simulink model "SVPWM1"  (Simulink 9.3)
settings: Solver=ode45  StartTime=0.0  StopTime=0.2  RelTol=1e-3
libraries: powerlib x12, simulink x1
settings Model: Creator=LENOVO  LastModifiedBy=LENOVO
settings DataIOCC: SaveFormat=Dataset  SignalLoggingSaveFormat=Dataset  ReturnWorkspaceOutputs=on
settings DebuggingCC: UnderspecifiedInitializationDetection=Simplified  MergeDetectMultiDrivingBlocksExec=error  FcnCallInpInsideContextMsg=error  SFUnexpectedBacktrackingDiag=error  SFNoUnconditionalDefaultTransitionDiag=error
settings HardwareCC: ProdBitPerPointer=64  ProdLargestAtomicFloat=Float  ProdIntDivRoundTo=Zero  ProdEndianess=LittleEndian  ProdHWDeviceType=Specified
settings ModelReferenceCC: PropagateSignalLabelsOutOfModel=on
settings SFSimCC: SimUseLocalCustomCode=on
settings RTWCC: RTWUseLocalCustomCode=on
settings GRTTargetCC: TargetLangStandard=C99 (ISO)  CombineOutputUpdateFcns=on  GRTInterface=off
settings ConfigComp: CovMetricSettings=dwe  CovHtmlReporting=off  CovSaveCumulativeToWorkspaceVar=off  CovSaveSingleToWorkspaceVar=off  CovExternalEMLEnable=on

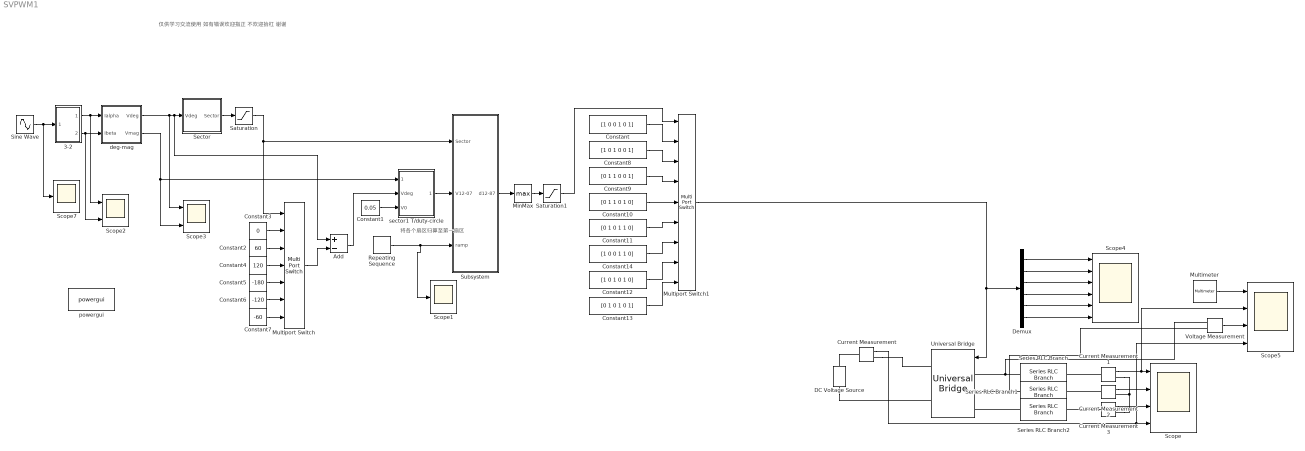
== system SVPWM1 ==
  note: 仅供学习交流使用 如有错误欢迎指正 不欢迎抬杠 谢谢
  note: 将各个扇区归算至第一扇区
  3-2 : Subsystem
  Add : Sum  Inputs=+-
  Constant : Constant  Value=[1 0 0 1 0 1]
  Constant1 : Constant  Value=0.05
  Constant10 : Constant  Value=[0 1 1 0 1 0]
  Constant11 : Constant  Value=[0 1 0 1 1 0]
  Constant12 : Constant  Value=[1 0 1 0 1 0]
  Constant13 : Constant  Value=[0 1 0 1 0 1]
  Constant14 : Constant  Value=[1 0 0 1 1 0]
  Constant2 : Constant  Value=60
  Constant3 : Constant  Value=0
  Constant4 : Constant  Value=120
  Constant5 : Constant  Value=-180
  Constant6 : Constant  Value=-120
  Constant7 : Constant  Value=-60
  Constant8 : Constant  Value=[1 0 1 0 0 1]
  Constant9 : Constant  Value=[0 1 1 0 0 1]
  Current Measurement{,1..3} (4 alike) : powerlib/Measurements/Current Measurement  PhasorSimulation=off  OutputType=Complex  PSBequivalent=0
      settings: SourceProductName=Simscape Electrical
  DC Voltage Source : powerlib/Electrical Sources/DC Voltage Source  Amplitude=100  Measurements=None
      settings: SourceProductName=Simscape Electrical
  Demux : Demux  Outputs=6
  MinMax : MinMax  Function=max
  Multimeter : powerlib/Measurements/Multimeter  PhasorSimulation=off  OutputType=Complex  sel=1  L=1  Gain=1  yselected={'Ub: Series RLC Branch'};  PSBOutputType=1  PSBequivalent=0  AxesSetting=[0,0.1,-100,100]  Display=0  SavedBlockNames=-11
      settings: SourceProductName=Simscape Electrical
  Multiport Switch : MultiPortSwitch  Inputs=6
  Multiport Switch1 : MultiPortSwitch  Inputs=8
  Repeating Sequence : simulink/Sources/Repeating Sequence  rep_seq_t=[0 1e-4]  rep_seq_y=[0 1]
  Saturation : Saturate  UpperLimit=6  LowerLimit=1
  Saturation1 : Saturate  UpperLimit=8  LowerLimit=1
  Scope : Scope  NumInputPorts=4
  Scope1 : Scope
  Scope2 : Scope  NumInputPorts=2
  Scope3 : Scope  NumInputPorts=2
  Scope4 : Scope  NumInputPorts=6
  Scope5 : Scope  NumInputPorts=4
  Scope7 : Scope
  Sector : Subsystem
  Series RLC Branch : powerlib/Elements/Series RLC Branch  LConnTagsString=__new0  RConnTagsString=__new0  BranchType=RL  Resistance=2  Inductance=5e-3  SetiL0=off  InitialCurrent=0  Capacitance=1e-6  Setx0=off  InitialVoltage=0  Measurements=Branch voltage
      settings: SourceProductName=Simscape Electrical
  Series RLC Branch1 : powerlib/Elements/Series RLC Branch  LConnTagsString=__new0  RConnTagsString=__new0  BranchType=RL  Resistance=2  Inductance=5e-3  SetiL0=off  InitialCurrent=0  Capacitance=1e-6  Setx0=off  InitialVoltage=0  Measurements=None
      settings: SourceProductName=Simscape Electrical
  Series RLC Branch2 : powerlib/Elements/Series RLC Branch  LConnTagsString=__new0  RConnTagsString=__new0  BranchType=RL  Resistance=2  Inductance=5e-3  SetiL0=off  InitialCurrent=0  Capacitance=1e-6  Setx0=off  InitialVoltage=0  Measurements=None
      settings: SourceProductName=Simscape Electrical
  Sine Wave : Sin  Amplitude=0.4  Frequency=2*pi*50  Phase=[0 -2*pi/3 2*pi/3]  SampleTime=1e-6
  Subsystem : Subsystem
  Universal Bridge : powerlib/Power Electronics/Universal Bridge  Arms=3  SnubberResistance=1e5  SnubberCapacitance=inf  Device=MOSFET / Diodes  Ron=1e-3  Lon=0  ForwardVoltages="[  0  0  ]"  ForwardVoltage=0  GTOparameters=[ 10e-6 , 20e-6 ]  IGBTparameters=[ 1e-6 , 2e-6 ]  Measurements=None  Measurements_2=None  converterType=Rectifier
      settings: SourceProductName=Simscape Electrical
  Voltage Measurement : powerlib/Measurements/Voltage Measurement  PhasorSimulation=off  OutputType=Complex  PSBequivalent=0
      settings: SourceProductName=Simscape Electrical
  deg-mag : Subsystem
  powergui : powerlib/powergui  Priority=1  SimulationMode=Continuous  SampleTime=50e-6  frequency=60  Iterations=50  frequencyindice=0  Pbase=100e6  ErrMax=1e-4  UnitsV=kV  UnitsW=MW  buscounter=0  FunctionMessages=off  echomessages=off  EnableUseOfTLC=off  CurrentSourceSwitches=off  DisableSnubberDevices=off  DisableRonSwitches=off  DisableVfSwitches=off  DisplayEquations=off  AutomaticDiscreteSolvers=off  SolverType=Tustin/Backward Euler (TBE)  Interpol=off  ExternalGateDelay=off  methode=off  Ts=100  x0status=blocks  SPID=on  SwTol=0  HookPort=off  NonlinearTolerance=0  nMaxIteration=15  ContinueOnMaxIteration=off  RestoreLinks=warning  ResistiveCurrentMeasurement=off  Frange=[0:2:500]  Ylog=off  Xlog=on  ShowGrid=off  save=off  variable=ZData  structure=0  ZoomFFT=off  StartTime=0.0  cycles=1  DisplayStyle=1  fundamental=60  FreqAxis=off  MaxFrequency=1000  frequencyindicesteady=1  RmsSteady=1  display=off
      settings: SourceProductName=Simscape Electrical
  sector1 T/duty-circle : Subsystem
  wires:
  Sine Wave/1 -> 3-2/1(Iabc), Scope7/1
  3-2/1(ialpha) -> deg-mag/1(Ialpha), Scope2/1
  3-2/2(ibeta) -> deg-mag/2(Ibeta), Scope2/2
  deg-mag/2(Vmag) -> Scope3/2, sector1 T/duty-circle/1(Vmag)
  Constant1/1 -> sector1 T/duty-circle/3(V0)
  Sector/1(Sector) -> Saturation/1
  Saturation/1 -> Multiport Switch/1, Subsystem/1("Sector ")
  deg-mag/1(Vdeg) -> Add/1, Sector/1(Vdeg), Scope3/1
  Constant2/1 -> Multiport Switch/3
  Constant3/1 -> Multiport Switch/2
  Constant5/1 -> Multiport Switch/5
  Constant6/1 -> Multiport Switch/6
  Constant7/1 -> Multiport Switch/7
  Constant4/1 -> Multiport Switch/4
  Multiport Switch/1 -> Add/2
  Repeating Sequence/1 -> Subsystem/3(ramp), Scope1/1
  sector1 T/duty-circle/1(V12-07) -> Subsystem/2(V12-07)
  Subsystem/1(d12-87) -> MinMax/1
  MinMax/1 -> Saturation1/1
  Saturation1/1 -> Multiport Switch1/1
  Constant/1 -> Multiport Switch1/2
  Constant8/1 -> Multiport Switch1/3
  Constant9/1 -> Multiport Switch1/4
  Constant13/1 -> Multiport Switch1/9
  Constant12/1 -> Multiport Switch1/8
  Constant14/1 -> Multiport Switch1/7
  Constant11/1 -> Multiport Switch1/6
  Constant10/1 -> Multiport Switch1/5
  Current Measurement/1 -> Scope5/4, Scope/4
  Multiport Switch1/1 -> Demux/1, Universal Bridge/1
  Current Measurement3/1 -> Scope/3
  Current Measurement1/1 -> Scope5/2, Scope/1
  Current Measurement2/1 -> Scope/2
  Demux/1 -> Scope4/1
  Demux/2 -> Scope4/2
  Demux/3 -> Scope4/3
  Demux/4 -> Scope4/4
  Demux/5 -> Scope4/5
  Demux/6 -> Scope4/6
  Add/1 -> sector1 T/duty-circle/2(Vdeg)
  Voltage Measurement/1 -> Scope5/3
  Multimeter/1 -> Scope5/1
  connections:
  Series RLC Branch1/LConn1 -- Voltage Measurement/LConn2 -- Universal Bridge/LConn2
  Series RLC Branch/LConn1 -- Voltage Measurement/LConn1 -- Universal Bridge/LConn1
  DC Voltage Source/LConn1 -- Universal Bridge/RConn2
  Series RLC Branch2/LConn1 -- Universal Bridge/LConn3
  Current Measurement/RConn1 -- Universal Bridge/RConn1
  Current Measurement/LConn1 -- DC Voltage Source/RConn1
  Current Measurement1/LConn1 -- Series RLC Branch/RConn1
  Current Measurement2/LConn1 -- Series RLC Branch1/RConn1
  Current Measurement3/LConn1 -- Series RLC Branch2/RConn1
  Current Measurement1/RConn1 -- Current Measurement3/RConn1 -- Current Measurement2/RConn1

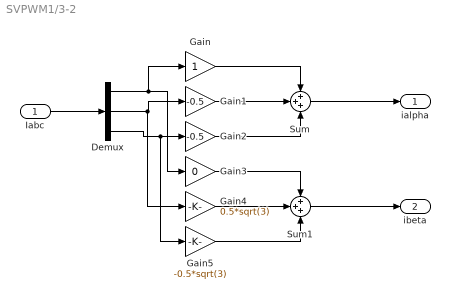
== system SVPWM1/3-2 ==
  Iabc : Inport
  Demux : Demux  Outputs=3
  Gain : Gain
  Gain1 : Gain  Gain=-0.5
  Gain2 : Gain  Gain=-0.5
  Gain3 : Gain  Gain=0
  Gain4 : Gain  Gain=0.5*sqrt(3)
  Gain5 : Gain  Gain=-0.5*sqrt(3)
  Sum : Sum  Inputs=+++
  Sum1 : Sum  Inputs=+++
  ialpha : Outport
  ibeta : Outport  Port=2
  wires:
  Gain2/1 -> Sum/3
  Gain1/1 -> Sum/2
  Gain4/1 -> Sum1/2
  Gain5/1 -> Sum1/3
  Demux/1 -> Gain3/1, Gain/1
  Gain/1 -> Sum/1
  Demux/2 -> Gain4/1, Gain1/1
  Demux/3 -> Gain5/1, Gain2/1
  Gain3/1 -> Sum1/1
  Sum/1 -> ialpha/1
  Sum1/1 -> ibeta/1
  Iabc/1 -> Demux/1

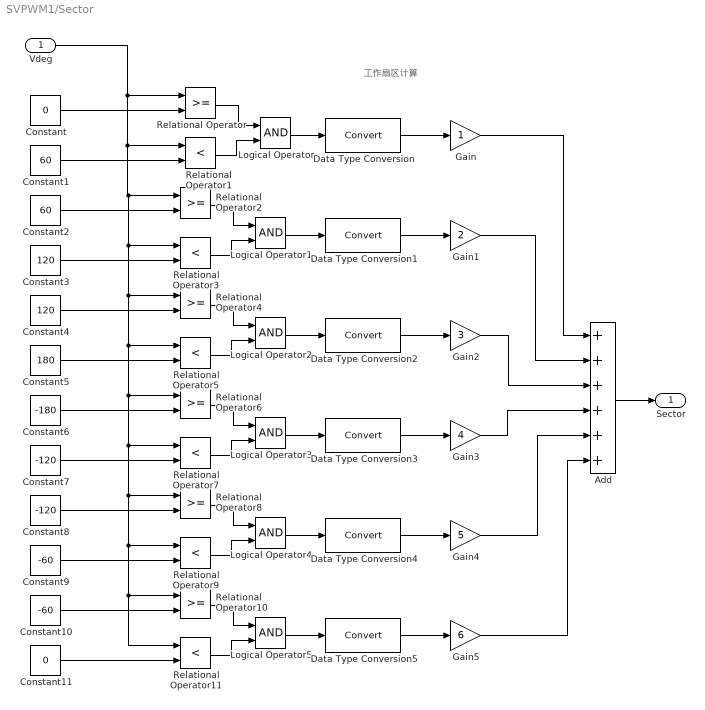
== system SVPWM1/Sector ==
  note: 工作扇区计算
  Vdeg : Inport
  Add : Sum  Inputs=++++++
  Constant : Constant  Value=0
  Constant1 : Constant  Value=60
  Constant10 : Constant  Value=-60
  Constant11 : Constant  Value=0
  Constant2 : Constant  Value=60
  Constant3 : Constant  Value=120
  Constant4 : Constant  Value=120
  Constant5 : Constant  Value=180
  Constant6 : Constant  Value=-180
  Constant7 : Constant  Value=-120
  Constant8 : Constant  Value=-120
  Constant9 : Constant  Value=-60
  Data Type Conversion{,1..5} (6 alike) : DataTypeConversion
  Gain : Gain
  Gain1 : Gain  Gain=2
  Gain2 : Gain  Gain=3
  Gain3 : Gain  Gain=4
  Gain4 : Gain  Gain=5
  Gain5 : Gain  Gain=6
  Logical Operator{,1..5} (6 alike) : Logic  AllPortsSameDT=off  OutDataTypeStr=boolean
  Relational Operator{,2,4,6,8,10} (6 alike) : RelationalOperator  OutDataTypeStr=boolean  RndMeth=Nearest
  Relational Operator{1,3,5,7,9,11} (6 alike) : RelationalOperator  Operator=<  OutDataTypeStr=boolean  RndMeth=Nearest
  Sector : Outport
  wires:
  Gain3/1 -> Add/4
  Logical Operator3/1 -> Data Type Conversion3/1
  Data Type Conversion3/1 -> Gain3/1
  Relational Operator/1 -> Logical Operator/1
  Data Type Conversion2/1 -> Gain2/1
  Relational Operator8/1 -> Logical Operator4/1
  Relational Operator5/1 -> Logical Operator2/2
  Vdeg/1 -> Relational Operator4/1, Relational Operator8/1, Relational Operator10/1, Relational Operator11/1, Relational Operator9/1, Relational Operator7/1, Relational Operator6/1, Relational Operator5/1, Relational Operator3/1, Relational Operator2/1, Relational Operator1/1, Relational Operator/1
  Constant2/1 -> Relational Operator2/2
  Data Type Conversion1/1 -> Gain1/1
  Constant1/1 -> Relational Operator1/2
  Relational Operator4/1 -> Logical Operator2/1
  Constant/1 -> Relational Operator/2
  Logical Operator/1 -> Data Type Conversion/1
  Gain2/1 -> Add/3
  Relational Operator3/1 -> Logical Operator1/2
  Relational Operator2/1 -> Logical Operator1/1
  Logical Operator1/1 -> Data Type Conversion1/1
  Constant10/1 -> Relational Operator10/2
  Relational Operator10/1 -> Logical Operator5/1
  Data Type Conversion5/1 -> Gain5/1
  Constant8/1 -> Relational Operator8/2
  Constant3/1 -> Relational Operator3/2
  Gain5/1 -> Add/6
  Relational Operator11/1 -> Logical Operator5/2
  Constant6/1 -> Relational Operator6/2
  Logical Operator5/1 -> Data Type Conversion5/1
  Logical Operator2/1 -> Data Type Conversion2/1
  Relational Operator6/1 -> Logical Operator3/1
  Data Type Conversion/1 -> Gain/1
  Constant11/1 -> Relational Operator11/2
  Gain1/1 -> Add/2
  Add/1 -> Sector/1
  Gain4/1 -> Add/5
  Constant4/1 -> Relational Operator4/2
  Constant5/1 -> Relational Operator5/2
  Relational Operator9/1 -> Logical Operator4/2
  Constant7/1 -> Relational Operator7/2
  Constant9/1 -> Relational Operator9/2
  Gain/1 -> Add/1
  Relational Operator1/1 -> Logical Operator/2
  Data Type Conversion4/1 -> Gain4/1
  Logical Operator4/1 -> Data Type Conversion4/1
  Relational Operator7/1 -> Logical Operator3/2

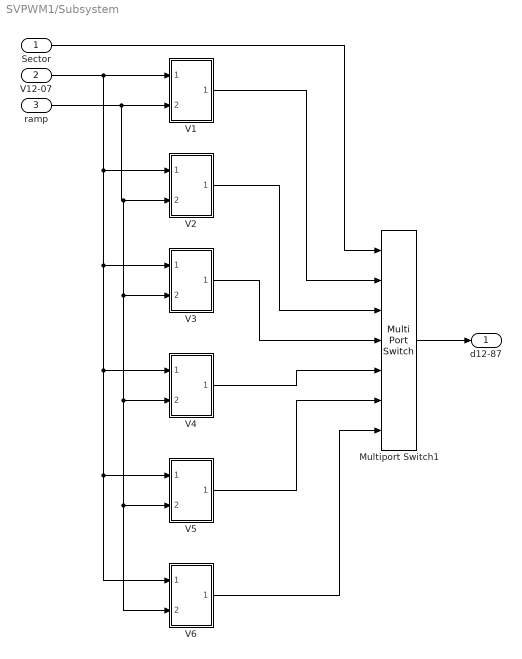
== system SVPWM1/Subsystem ==
  "Sector " : Inport
  V12-07 : Inport  Port=2
  ramp : Inport  Port=3
  Multiport Switch1 : MultiPortSwitch  Inputs=6
  "V1 " : Subsystem
  V2 : Subsystem
  V3 : Subsystem
  V4 : Subsystem
  V5 : Subsystem
  V6 : Subsystem
  d12-87 : Outport
  wires:
  V12-07/1 -> V6/1(V12-07), V5/1(V12-07), V4/1(V12-07), V3/1(V12-07), V2/1(V12-07), "V1 "/1(V12-07)
  Multiport Switch1/1 -> d12-87/1
  V2/1(Output) -> Multiport Switch1/3
  "V1 "/1(Output) -> Multiport Switch1/2
  V3/1(Output) -> Multiport Switch1/4
  V6/1(Output) -> Multiport Switch1/7
  ramp/1 -> V5/2(ramp), V6/2(ramp), V4/2(ramp), V3/2(ramp), V2/2(ramp), "V1 "/2(ramp)
  V4/1(Output) -> Multiport Switch1/5
  V5/1(Output) -> Multiport Switch1/6
  "Sector "/1 -> Multiport Switch1/1

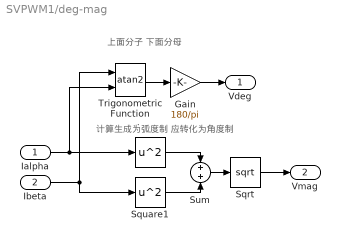
== system SVPWM1/deg-mag ==
  note: 计算生成为弧度制 应转化为角度制
  note: 上面分子 下面分母
  Ialpha : Inport
  Ibeta : Inport  Port=2
  Gain : Gain  Gain=180/pi
  Sqrt : Sqrt  SaturateOnIntegerOverflow=on
  Square : Math  Operator=square  SaturateOnIntegerOverflow=on
  Square1 : Math  Operator=square  SaturateOnIntegerOverflow=on
  Sum : Sum  Inputs=+|+
  Trigonometric Function : Trigonometry  Operator=atan2
  Vdeg : Outport
  Vmag : Outport  Port=2
  wires:
  Ibeta/1 -> Square1/1, Trigonometric Function/1
  Gain/1 -> Vdeg/1
  Trigonometric Function/1 -> Gain/1
  Ialpha/1 -> Trigonometric Function/2, Square/1
  Sum/1 -> Sqrt/1
  Square/1 -> Sum/1
  Square1/1 -> Sum/2
  Sqrt/1 -> Vmag/1

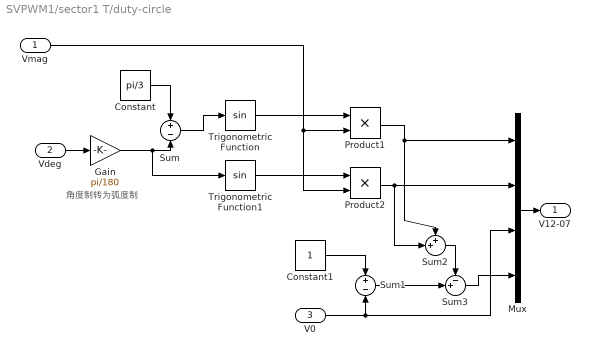
== system SVPWM1/sector1 T/duty-circle ==
  note: 角度制转为弧度制
  Vmag : Inport
  Vdeg : Inport  Port=2
  V0 : Inport  Port=3
  Constant : Constant  Value=pi/3
  Constant1 : Constant
  Gain : Gain  Gain=pi/180
  Mux : Mux
  Product1 : Product
  Product2 : Product
  Sum : Sum  Inputs=+|-
  Sum1 : Sum  Inputs=+|-
  Sum2 : Sum  Inputs=++|
  Sum3 : Sum  Inputs=-+|
  Trigonometric Function : Trigonometry
  Trigonometric Function1 : Trigonometry
  V12-07 : Outport
  wires:
  Trigonometric Function/1 -> Product1/1
  Trigonometric Function1/1 -> Product2/1
  Gain/1 -> Trigonometric Function1/1, Sum/2
  Product2/1 -> Sum2/2, Mux/2
  Sum/1 -> Trigonometric Function/1
  Product1/1 -> Mux/1, Sum2/1
  Constant/1 -> Sum/1
  Constant1/1 -> Sum1/1
  Sum2/1 -> Sum3/1
  Sum1/1 -> Sum3/2
  Mux/1 -> V12-07/1
  V0/1 -> Mux/3, Sum1/2
  Sum3/1 -> Mux/4
  Vdeg/1 -> Gain/1
  Vmag/1 -> Product2/2, Product1/2

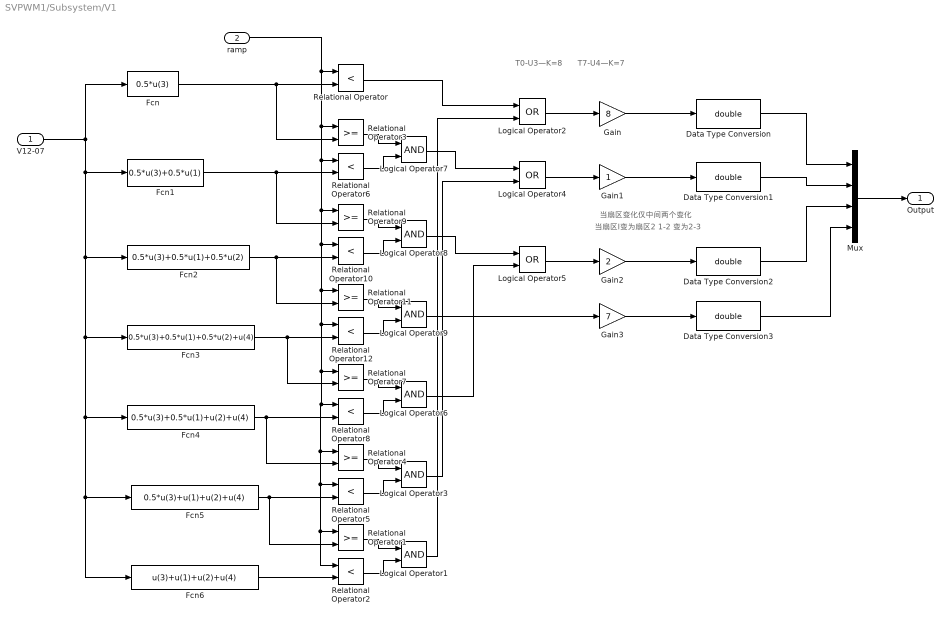
== system SVPWM1/Subsystem/V1  ==
  note: 当扇区I变为扇区2 1-2 变为2-3
  note: 当扇区变化仅中间两个变化
  note: T7-U4—K=7
  note: T0-U3—K=8
  V12-07 : Inport
  ramp : Inport  Port=2
  Data Type Conversion{,1..3} (4 alike) : DataTypeConversion  OutDataTypeStr=double
  Fcn : Fcn  Expr=0.5*u(3)
  Fcn1 : Fcn  Expr=0.5*u(3)+0.5*u(1)
  Fcn2 : Fcn  Expr=0.5*u(3)+0.5*u(1)+0.5*u(2)
  Fcn3 : Fcn  Expr=0.5*u(3)+0.5*u(1)+0.5*u(2)+u(4)
  Fcn4 : Fcn  Expr=0.5*u(3)+0.5*u(1)+u(2)+u(4)
  Fcn5 : Fcn  Expr=0.5*u(3)+u(1)+u(2)+u(4)
  Fcn6 : Fcn  Expr=u(3)+u(1)+u(2)+u(4)
  Gain : Gain  Gain=8
  Gain1 : Gain
  Gain2 : Gain  Gain=2
  Gain3 : Gain  Gain=7
  Logical Operator{1,3,6..9} (6 alike) : Logic  AllPortsSameDT=off  OutDataTypeStr=boolean
  Logical Operator2 : Logic  Operator=OR  AllPortsSameDT=off  OutDataTypeStr=boolean
  Logical Operator4 : Logic  Operator=OR  AllPortsSameDT=off  OutDataTypeStr=boolean
  Logical Operator5 : Logic  Operator=OR  AllPortsSameDT=off  OutDataTypeStr=boolean
  Mux : Mux
  Relational Operator{,2,5..6,8,10,12} (7 alike) : RelationalOperator  Operator=<  OutDataTypeStr=boolean  RndMeth=Nearest
  Relational Operator{1,3..4,7,9,11} (6 alike) : RelationalOperator  OutDataTypeStr=boolean  RndMeth=Nearest
  Output : Outport
  wires:
  Relational Operator8/1 -> Logical Operator6/2
  Relational Operator12/1 -> Logical Operator9/2
  ramp/1 -> Relational Operator11/1, Relational Operator12/1, Relational Operator5/1, Relational Operator1/1, Relational Operator2/1, Relational Operator4/1, Relational Operator8/1, Relational Operator7/1, Relational Operator10/1, Relational Operator9/1, Relational Operator6/1, Relational Operator3/1, Relational Operator/1
  Fcn/1 -> Relational Operator3/2, Relational Operator/2
  Relational Operator5/1 -> Logical Operator3/2
  Data Type Conversion3/1 -> Mux/4
  Logical Operator4/1 -> Gain1/1
  Relational Operator11/1 -> Logical Operator9/1
  Logical Operator6/1 -> Logical Operator5/2
  Logical Operator8/1 -> Logical Operator5/1
  Relational Operator4/1 -> Logical Operator3/1
  Relational Operator9/1 -> Logical Operator8/1
  Logical Operator1/1 -> Logical Operator2/2
  Logical Operator5/1 -> Gain2/1
  Data Type Conversion1/1 -> Mux/2
  Fcn1/1 -> Relational Operator9/2, Relational Operator6/2
  Fcn3/1 -> Relational Operator12/2, Relational Operator7/2
  Logical Operator3/1 -> Logical Operator4/2
  Fcn4/1 -> Relational Operator8/2, Relational Operator4/2
  Fcn6/1 -> Relational Operator2/2
  Gain2/1 -> Data Type Conversion2/1
  Logical Operator2/1 -> Gain/1
  V12-07/1 -> Fcn1/1, Fcn4/1, Fcn6/1, Fcn5/1, Fcn3/1, Fcn2/1, Fcn/1
  Fcn2/1 -> Relational Operator11/2, Relational Operator10/2
  Fcn5/1 -> Relational Operator5/2, Relational Operator1/2
  Gain3/1 -> Data Type Conversion3/1
  Mux/1 -> Output/1
  Data Type Conversion2/1 -> Mux/3
  Relational Operator7/1 -> Logical Operator6/1
  Data Type Conversion/1 -> Mux/1
  Relational Operator6/1 -> Logical Operator7/2
  Relational Operator3/1 -> Logical Operator7/1
  Logical Operator7/1 -> Logical Operator4/1
  Relational Operator10/1 -> Logical Operator8/2
  Gain1/1 -> Data Type Conversion1/1
  Logical Operator9/1 -> Gain3/1
  Relational Operator/1 -> Logical Operator2/1
  Relational Operator1/1 -> Logical Operator1/1
  Relational Operator2/1 -> Logical Operator1/2
  Gain/1 -> Data Type Conversion/1

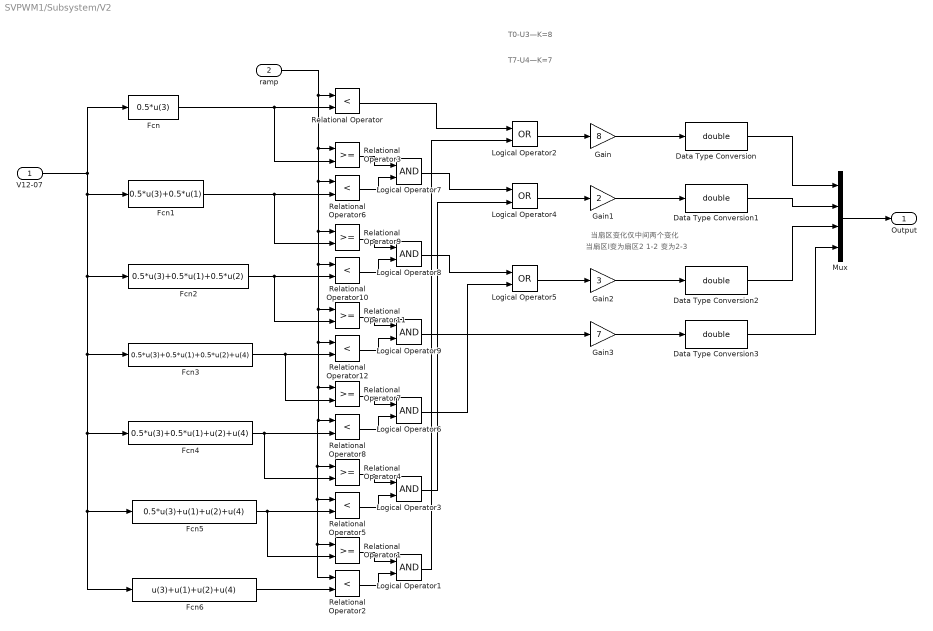
== system SVPWM1/Subsystem/V2 ==
  note: 当扇区I变为扇区2 1-2 变为2-3
  note: 当扇区变化仅中间两个变化
  note: T7-U4—K=7
  note: T0-U3—K=8
  V12-07 : Inport
  ramp : Inport  Port=2
  Data Type Conversion{,1..3} (4 alike) : DataTypeConversion  OutDataTypeStr=double
  Fcn : Fcn  Expr=0.5*u(3)
  Fcn1 : Fcn  Expr=0.5*u(3)+0.5*u(1)
  Fcn2 : Fcn  Expr=0.5*u(3)+0.5*u(1)+0.5*u(2)
  Fcn3 : Fcn  Expr=0.5*u(3)+0.5*u(1)+0.5*u(2)+u(4)
  Fcn4 : Fcn  Expr=0.5*u(3)+0.5*u(1)+u(2)+u(4)
  Fcn5 : Fcn  Expr=0.5*u(3)+u(1)+u(2)+u(4)
  Fcn6 : Fcn  Expr=u(3)+u(1)+u(2)+u(4)
  Gain : Gain  Gain=8
  Gain1 : Gain  Gain=2
  Gain2 : Gain  Gain=3
  Gain3 : Gain  Gain=7
  Logical Operator{1,3,6..9} (6 alike) : Logic  AllPortsSameDT=off  OutDataTypeStr=boolean
  Logical Operator2 : Logic  Operator=OR  AllPortsSameDT=off  OutDataTypeStr=boolean
  Logical Operator4 : Logic  Operator=OR  AllPortsSameDT=off  OutDataTypeStr=boolean
  Logical Operator5 : Logic  Operator=OR  AllPortsSameDT=off  OutDataTypeStr=boolean
  Mux : Mux
  Relational Operator{,2,5..6,8,10,12} (7 alike) : RelationalOperator  Operator=<  OutDataTypeStr=boolean  RndMeth=Nearest
  Relational Operator{1,3..4,7,9,11} (6 alike) : RelationalOperator  OutDataTypeStr=boolean  RndMeth=Nearest
  Output : Outport
  wires:
  Relational Operator8/1 -> Logical Operator6/2
  Relational Operator12/1 -> Logical Operator9/2
  ramp/1 -> Relational Operator11/1, Relational Operator12/1, Relational Operator5/1, Relational Operator1/1, Relational Operator2/1, Relational Operator4/1, Relational Operator8/1, Relational Operator7/1, Relational Operator10/1, Relational Operator9/1, Relational Operator6/1, Relational Operator3/1, Relational Operator/1
  Fcn/1 -> Relational Operator3/2, Relational Operator/2
  Relational Operator5/1 -> Logical Operator3/2
  Data Type Conversion3/1 -> Mux/4
  Logical Operator4/1 -> Gain1/1
  Relational Operator11/1 -> Logical Operator9/1
  Logical Operator6/1 -> Logical Operator5/2
  Logical Operator8/1 -> Logical Operator5/1
  Relational Operator4/1 -> Logical Operator3/1
  Relational Operator9/1 -> Logical Operator8/1
  Logical Operator1/1 -> Logical Operator2/2
  Logical Operator5/1 -> Gain2/1
  Data Type Conversion1/1 -> Mux/2
  Fcn1/1 -> Relational Operator9/2, Relational Operator6/2
  Fcn3/1 -> Relational Operator12/2, Relational Operator7/2
  Logical Operator3/1 -> Logical Operator4/2
  Fcn4/1 -> Relational Operator8/2, Relational Operator4/2
  Fcn6/1 -> Relational Operator2/2
  Gain2/1 -> Data Type Conversion2/1
  Logical Operator2/1 -> Gain/1
  V12-07/1 -> Fcn1/1, Fcn4/1, Fcn6/1, Fcn5/1, Fcn3/1, Fcn2/1, Fcn/1
  Fcn2/1 -> Relational Operator11/2, Relational Operator10/2
  Fcn5/1 -> Relational Operator5/2, Relational Operator1/2
  Gain3/1 -> Data Type Conversion3/1
  Mux/1 -> Output/1
  Data Type Conversion2/1 -> Mux/3
  Relational Operator7/1 -> Logical Operator6/1
  Data Type Conversion/1 -> Mux/1
  Relational Operator6/1 -> Logical Operator7/2
  Relational Operator3/1 -> Logical Operator7/1
  Logical Operator7/1 -> Logical Operator4/1
  Relational Operator10/1 -> Logical Operator8/2
  Gain1/1 -> Data Type Conversion1/1
  Logical Operator9/1 -> Gain3/1
  Relational Operator/1 -> Logical Operator2/1
  Relational Operator1/1 -> Logical Operator1/1
  Relational Operator2/1 -> Logical Operator1/2
  Gain/1 -> Data Type Conversion/1

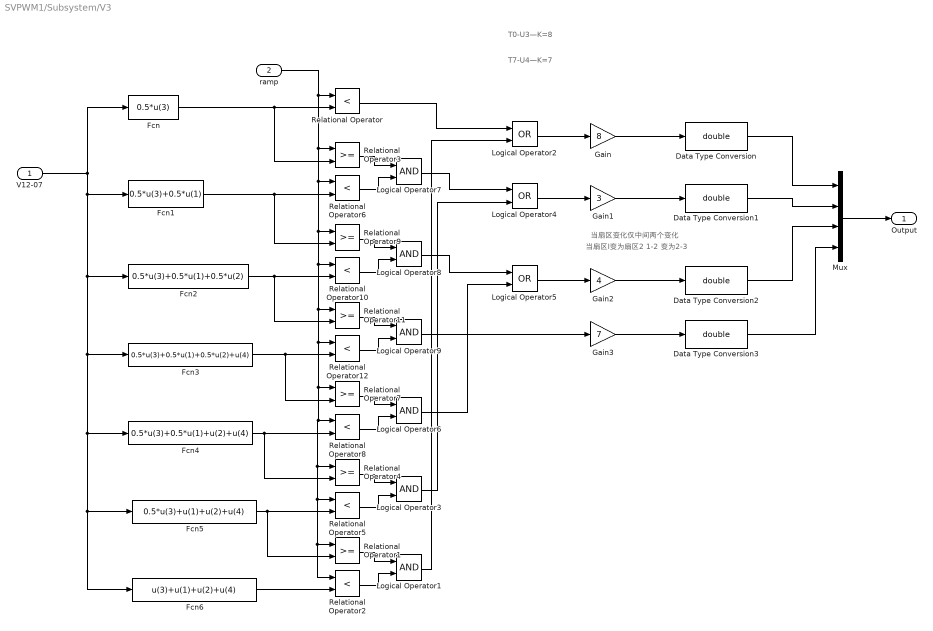
== system SVPWM1/Subsystem/V3 ==
  note: 当扇区I变为扇区2 1-2 变为2-3
  note: 当扇区变化仅中间两个变化
  note: T7-U4—K=7
  note: T0-U3—K=8
  V12-07 : Inport
  ramp : Inport  Port=2
  Data Type Conversion{,1..3} (4 alike) : DataTypeConversion  OutDataTypeStr=double
  Fcn : Fcn  Expr=0.5*u(3)
  Fcn1 : Fcn  Expr=0.5*u(3)+0.5*u(1)
  Fcn2 : Fcn  Expr=0.5*u(3)+0.5*u(1)+0.5*u(2)
  Fcn3 : Fcn  Expr=0.5*u(3)+0.5*u(1)+0.5*u(2)+u(4)
  Fcn4 : Fcn  Expr=0.5*u(3)+0.5*u(1)+u(2)+u(4)
  Fcn5 : Fcn  Expr=0.5*u(3)+u(1)+u(2)+u(4)
  Fcn6 : Fcn  Expr=u(3)+u(1)+u(2)+u(4)
  Gain : Gain  Gain=8
  Gain1 : Gain  Gain=3
  Gain2 : Gain  Gain=4
  Gain3 : Gain  Gain=7
  Logical Operator{1,3,6..9} (6 alike) : Logic  AllPortsSameDT=off  OutDataTypeStr=boolean
  Logical Operator2 : Logic  Operator=OR  AllPortsSameDT=off  OutDataTypeStr=boolean
  Logical Operator4 : Logic  Operator=OR  AllPortsSameDT=off  OutDataTypeStr=boolean
  Logical Operator5 : Logic  Operator=OR  AllPortsSameDT=off  OutDataTypeStr=boolean
  Mux : Mux
  Relational Operator{,2,5..6,8,10,12} (7 alike) : RelationalOperator  Operator=<  OutDataTypeStr=boolean  RndMeth=Nearest
  Relational Operator{1,3..4,7,9,11} (6 alike) : RelationalOperator  OutDataTypeStr=boolean  RndMeth=Nearest
  Output : Outport
  wires:
  Relational Operator8/1 -> Logical Operator6/2
  Relational Operator12/1 -> Logical Operator9/2
  ramp/1 -> Relational Operator11/1, Relational Operator12/1, Relational Operator5/1, Relational Operator1/1, Relational Operator2/1, Relational Operator4/1, Relational Operator8/1, Relational Operator7/1, Relational Operator10/1, Relational Operator9/1, Relational Operator6/1, Relational Operator3/1, Relational Operator/1
  Fcn/1 -> Relational Operator3/2, Relational Operator/2
  Relational Operator5/1 -> Logical Operator3/2
  Data Type Conversion3/1 -> Mux/4
  Logical Operator4/1 -> Gain1/1
  Relational Operator11/1 -> Logical Operator9/1
  Logical Operator6/1 -> Logical Operator5/2
  Logical Operator8/1 -> Logical Operator5/1
  Relational Operator4/1 -> Logical Operator3/1
  Relational Operator9/1 -> Logical Operator8/1
  Logical Operator1/1 -> Logical Operator2/2
  Logical Operator5/1 -> Gain2/1
  Data Type Conversion1/1 -> Mux/2
  Fcn1/1 -> Relational Operator9/2, Relational Operator6/2
  Fcn3/1 -> Relational Operator12/2, Relational Operator7/2
  Logical Operator3/1 -> Logical Operator4/2
  Fcn4/1 -> Relational Operator8/2, Relational Operator4/2
  Fcn6/1 -> Relational Operator2/2
  Gain2/1 -> Data Type Conversion2/1
  Logical Operator2/1 -> Gain/1
  V12-07/1 -> Fcn1/1, Fcn4/1, Fcn6/1, Fcn5/1, Fcn3/1, Fcn2/1, Fcn/1
  Fcn2/1 -> Relational Operator11/2, Relational Operator10/2
  Fcn5/1 -> Relational Operator5/2, Relational Operator1/2
  Gain3/1 -> Data Type Conversion3/1
  Mux/1 -> Output/1
  Data Type Conversion2/1 -> Mux/3
  Relational Operator7/1 -> Logical Operator6/1
  Data Type Conversion/1 -> Mux/1
  Relational Operator6/1 -> Logical Operator7/2
  Relational Operator3/1 -> Logical Operator7/1
  Logical Operator7/1 -> Logical Operator4/1
  Relational Operator10/1 -> Logical Operator8/2
  Gain1/1 -> Data Type Conversion1/1
  Logical Operator9/1 -> Gain3/1
  Relational Operator/1 -> Logical Operator2/1
  Relational Operator1/1 -> Logical Operator1/1
  Relational Operator2/1 -> Logical Operator1/2
  Gain/1 -> Data Type Conversion/1

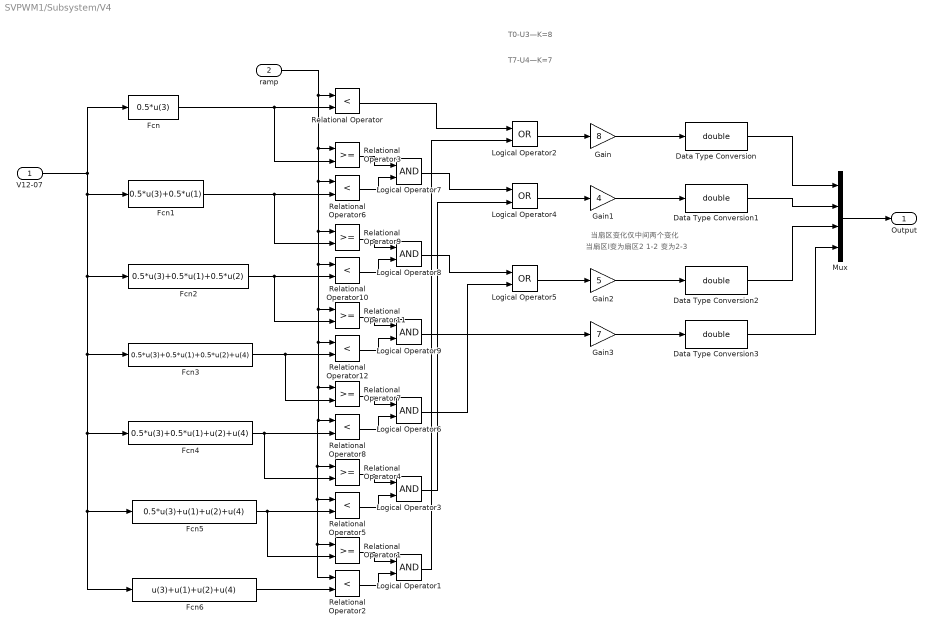
== system SVPWM1/Subsystem/V4 ==
  note: 当扇区I变为扇区2 1-2 变为2-3
  note: 当扇区变化仅中间两个变化
  note: T7-U4—K=7
  note: T0-U3—K=8
  V12-07 : Inport
  ramp : Inport  Port=2
  Data Type Conversion{,1..3} (4 alike) : DataTypeConversion  OutDataTypeStr=double
  Fcn : Fcn  Expr=0.5*u(3)
  Fcn1 : Fcn  Expr=0.5*u(3)+0.5*u(1)
  Fcn2 : Fcn  Expr=0.5*u(3)+0.5*u(1)+0.5*u(2)
  Fcn3 : Fcn  Expr=0.5*u(3)+0.5*u(1)+0.5*u(2)+u(4)
  Fcn4 : Fcn  Expr=0.5*u(3)+0.5*u(1)+u(2)+u(4)
  Fcn5 : Fcn  Expr=0.5*u(3)+u(1)+u(2)+u(4)
  Fcn6 : Fcn  Expr=u(3)+u(1)+u(2)+u(4)
  Gain : Gain  Gain=8
  Gain1 : Gain  Gain=4
  Gain2 : Gain  Gain=5
  Gain3 : Gain  Gain=7
  Logical Operator{1,3,6..9} (6 alike) : Logic  AllPortsSameDT=off  OutDataTypeStr=boolean
  Logical Operator2 : Logic  Operator=OR  AllPortsSameDT=off  OutDataTypeStr=boolean
  Logical Operator4 : Logic  Operator=OR  AllPortsSameDT=off  OutDataTypeStr=boolean
  Logical Operator5 : Logic  Operator=OR  AllPortsSameDT=off  OutDataTypeStr=boolean
  Mux : Mux
  Relational Operator{,2,5..6,8,10,12} (7 alike) : RelationalOperator  Operator=<  OutDataTypeStr=boolean  RndMeth=Nearest
  Relational Operator{1,3..4,7,9,11} (6 alike) : RelationalOperator  OutDataTypeStr=boolean  RndMeth=Nearest
  Output : Outport
  wires:
  Relational Operator8/1 -> Logical Operator6/2
  Relational Operator12/1 -> Logical Operator9/2
  ramp/1 -> Relational Operator11/1, Relational Operator12/1, Relational Operator5/1, Relational Operator1/1, Relational Operator2/1, Relational Operator4/1, Relational Operator8/1, Relational Operator7/1, Relational Operator10/1, Relational Operator9/1, Relational Operator6/1, Relational Operator3/1, Relational Operator/1
  Fcn/1 -> Relational Operator3/2, Relational Operator/2
  Relational Operator5/1 -> Logical Operator3/2
  Data Type Conversion3/1 -> Mux/4
  Logical Operator4/1 -> Gain1/1
  Relational Operator11/1 -> Logical Operator9/1
  Logical Operator6/1 -> Logical Operator5/2
  Logical Operator8/1 -> Logical Operator5/1
  Relational Operator4/1 -> Logical Operator3/1
  Relational Operator9/1 -> Logical Operator8/1
  Logical Operator1/1 -> Logical Operator2/2
  Logical Operator5/1 -> Gain2/1
  Data Type Conversion1/1 -> Mux/2
  Fcn1/1 -> Relational Operator9/2, Relational Operator6/2
  Fcn3/1 -> Relational Operator12/2, Relational Operator7/2
  Logical Operator3/1 -> Logical Operator4/2
  Fcn4/1 -> Relational Operator8/2, Relational Operator4/2
  Fcn6/1 -> Relational Operator2/2
  Gain2/1 -> Data Type Conversion2/1
  Logical Operator2/1 -> Gain/1
  V12-07/1 -> Fcn1/1, Fcn4/1, Fcn6/1, Fcn5/1, Fcn3/1, Fcn2/1, Fcn/1
  Fcn2/1 -> Relational Operator11/2, Relational Operator10/2
  Fcn5/1 -> Relational Operator5/2, Relational Operator1/2
  Gain3/1 -> Data Type Conversion3/1
  Mux/1 -> Output/1
  Data Type Conversion2/1 -> Mux/3
  Relational Operator7/1 -> Logical Operator6/1
  Data Type Conversion/1 -> Mux/1
  Relational Operator6/1 -> Logical Operator7/2
  Relational Operator3/1 -> Logical Operator7/1
  Logical Operator7/1 -> Logical Operator4/1
  Relational Operator10/1 -> Logical Operator8/2
  Gain1/1 -> Data Type Conversion1/1
  Logical Operator9/1 -> Gain3/1
  Relational Operator/1 -> Logical Operator2/1
  Relational Operator1/1 -> Logical Operator1/1
  Relational Operator2/1 -> Logical Operator1/2
  Gain/1 -> Data Type Conversion/1

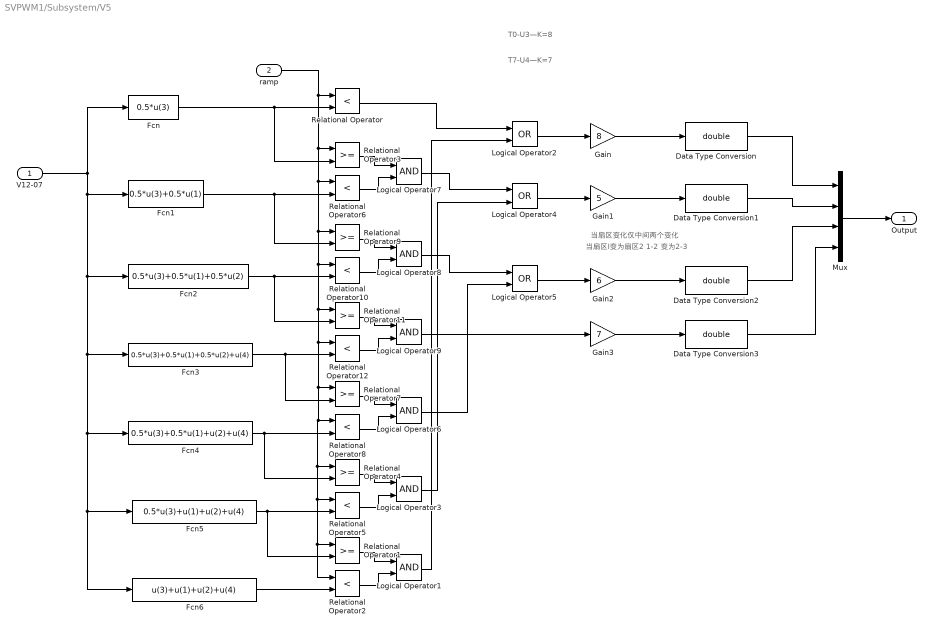
== system SVPWM1/Subsystem/V5 ==
  note: 当扇区I变为扇区2 1-2 变为2-3
  note: 当扇区变化仅中间两个变化
  note: T7-U4—K=7
  note: T0-U3—K=8
  V12-07 : Inport
  ramp : Inport  Port=2
  Data Type Conversion{,1..3} (4 alike) : DataTypeConversion  OutDataTypeStr=double
  Fcn : Fcn  Expr=0.5*u(3)
  Fcn1 : Fcn  Expr=0.5*u(3)+0.5*u(1)
  Fcn2 : Fcn  Expr=0.5*u(3)+0.5*u(1)+0.5*u(2)
  Fcn3 : Fcn  Expr=0.5*u(3)+0.5*u(1)+0.5*u(2)+u(4)
  Fcn4 : Fcn  Expr=0.5*u(3)+0.5*u(1)+u(2)+u(4)
  Fcn5 : Fcn  Expr=0.5*u(3)+u(1)+u(2)+u(4)
  Fcn6 : Fcn  Expr=u(3)+u(1)+u(2)+u(4)
  Gain : Gain  Gain=8
  Gain1 : Gain  Gain=5
  Gain2 : Gain  Gain=6
  Gain3 : Gain  Gain=7
  Logical Operator{1,3,6..9} (6 alike) : Logic  AllPortsSameDT=off  OutDataTypeStr=boolean
  Logical Operator2 : Logic  Operator=OR  AllPortsSameDT=off  OutDataTypeStr=boolean
  Logical Operator4 : Logic  Operator=OR  AllPortsSameDT=off  OutDataTypeStr=boolean
  Logical Operator5 : Logic  Operator=OR  AllPortsSameDT=off  OutDataTypeStr=boolean
  Mux : Mux
  Relational Operator{,2,5..6,8,10,12} (7 alike) : RelationalOperator  Operator=<  OutDataTypeStr=boolean  RndMeth=Nearest
  Relational Operator{1,3..4,7,9,11} (6 alike) : RelationalOperator  OutDataTypeStr=boolean  RndMeth=Nearest
  Output : Outport
  wires:
  Relational Operator8/1 -> Logical Operator6/2
  Relational Operator12/1 -> Logical Operator9/2
  ramp/1 -> Relational Operator11/1, Relational Operator12/1, Relational Operator5/1, Relational Operator1/1, Relational Operator2/1, Relational Operator4/1, Relational Operator8/1, Relational Operator7/1, Relational Operator10/1, Relational Operator9/1, Relational Operator6/1, Relational Operator3/1, Relational Operator/1
  Fcn/1 -> Relational Operator3/2, Relational Operator/2
  Relational Operator5/1 -> Logical Operator3/2
  Data Type Conversion3/1 -> Mux/4
  Logical Operator4/1 -> Gain1/1
  Relational Operator11/1 -> Logical Operator9/1
  Logical Operator6/1 -> Logical Operator5/2
  Logical Operator8/1 -> Logical Operator5/1
  Relational Operator4/1 -> Logical Operator3/1
  Relational Operator9/1 -> Logical Operator8/1
  Logical Operator1/1 -> Logical Operator2/2
  Logical Operator5/1 -> Gain2/1
  Data Type Conversion1/1 -> Mux/2
  Fcn1/1 -> Relational Operator9/2, Relational Operator6/2
  Fcn3/1 -> Relational Operator12/2, Relational Operator7/2
  Logical Operator3/1 -> Logical Operator4/2
  Fcn4/1 -> Relational Operator8/2, Relational Operator4/2
  Fcn6/1 -> Relational Operator2/2
  Gain2/1 -> Data Type Conversion2/1
  Logical Operator2/1 -> Gain/1
  V12-07/1 -> Fcn1/1, Fcn4/1, Fcn6/1, Fcn5/1, Fcn3/1, Fcn2/1, Fcn/1
  Fcn2/1 -> Relational Operator11/2, Relational Operator10/2
  Fcn5/1 -> Relational Operator5/2, Relational Operator1/2
  Gain3/1 -> Data Type Conversion3/1
  Mux/1 -> Output/1
  Data Type Conversion2/1 -> Mux/3
  Relational Operator7/1 -> Logical Operator6/1
  Data Type Conversion/1 -> Mux/1
  Relational Operator6/1 -> Logical Operator7/2
  Relational Operator3/1 -> Logical Operator7/1
  Logical Operator7/1 -> Logical Operator4/1
  Relational Operator10/1 -> Logical Operator8/2
  Gain1/1 -> Data Type Conversion1/1
  Logical Operator9/1 -> Gain3/1
  Relational Operator/1 -> Logical Operator2/1
  Relational Operator1/1 -> Logical Operator1/1
  Relational Operator2/1 -> Logical Operator1/2
  Gain/1 -> Data Type Conversion/1

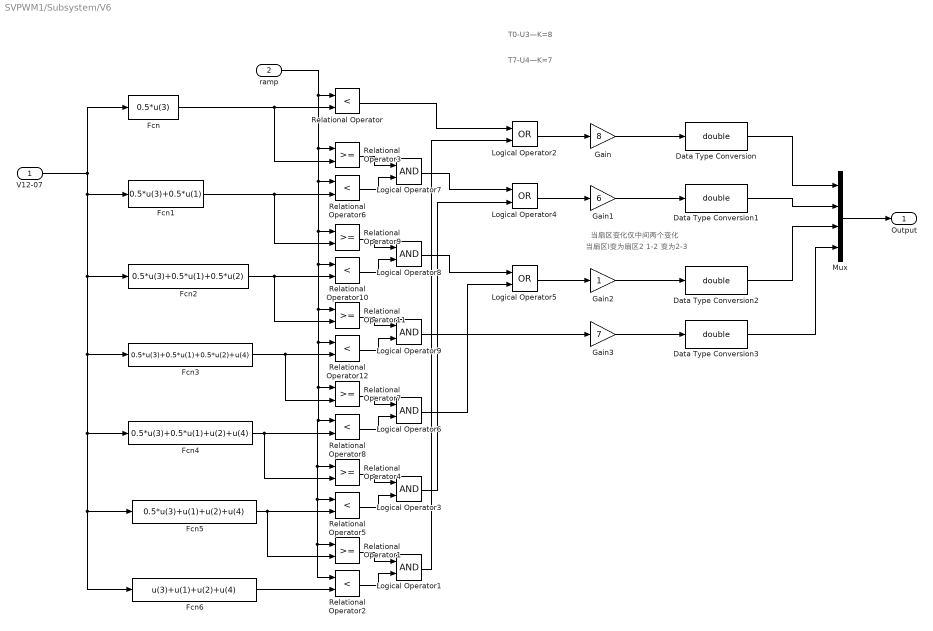
== system SVPWM1/Subsystem/V6 ==
  note: 当扇区I变为扇区2 1-2 变为2-3
  note: 当扇区变化仅中间两个变化
  note: T7-U4—K=7
  note: T0-U3—K=8
  V12-07 : Inport
  ramp : Inport  Port=2
  Data Type Conversion{,1..3} (4 alike) : DataTypeConversion  OutDataTypeStr=double
  Fcn : Fcn  Expr=0.5*u(3)
  Fcn1 : Fcn  Expr=0.5*u(3)+0.5*u(1)
  Fcn2 : Fcn  Expr=0.5*u(3)+0.5*u(1)+0.5*u(2)
  Fcn3 : Fcn  Expr=0.5*u(3)+0.5*u(1)+0.5*u(2)+u(4)
  Fcn4 : Fcn  Expr=0.5*u(3)+0.5*u(1)+u(2)+u(4)
  Fcn5 : Fcn  Expr=0.5*u(3)+u(1)+u(2)+u(4)
  Fcn6 : Fcn  Expr=u(3)+u(1)+u(2)+u(4)
  Gain : Gain  Gain=8
  Gain1 : Gain  Gain=6
  Gain2 : Gain
  Gain3 : Gain  Gain=7
  Logical Operator{1,3,6..9} (6 alike) : Logic  AllPortsSameDT=off  OutDataTypeStr=boolean
  Logical Operator2 : Logic  Operator=OR  AllPortsSameDT=off  OutDataTypeStr=boolean
  Logical Operator4 : Logic  Operator=OR  AllPortsSameDT=off  OutDataTypeStr=boolean
  Logical Operator5 : Logic  Operator=OR  AllPortsSameDT=off  OutDataTypeStr=boolean
  Mux : Mux
  Relational Operator{,2,5..6,8,10,12} (7 alike) : RelationalOperator  Operator=<  OutDataTypeStr=boolean  RndMeth=Nearest
  Relational Operator{1,3..4,7,9,11} (6 alike) : RelationalOperator  OutDataTypeStr=boolean  RndMeth=Nearest
  Output : Outport
  wires:
  Relational Operator8/1 -> Logical Operator6/2
  Relational Operator12/1 -> Logical Operator9/2
  ramp/1 -> Relational Operator11/1, Relational Operator12/1, Relational Operator5/1, Relational Operator1/1, Relational Operator2/1, Relational Operator4/1, Relational Operator8/1, Relational Operator7/1, Relational Operator10/1, Relational Operator9/1, Relational Operator6/1, Relational Operator3/1, Relational Operator/1
  Fcn/1 -> Relational Operator3/2, Relational Operator/2
  Relational Operator5/1 -> Logical Operator3/2
  Data Type Conversion3/1 -> Mux/4
  Logical Operator4/1 -> Gain1/1
  Relational Operator11/1 -> Logical Operator9/1
  Logical Operator6/1 -> Logical Operator5/2
  Logical Operator8/1 -> Logical Operator5/1
  Relational Operator4/1 -> Logical Operator3/1
  Relational Operator9/1 -> Logical Operator8/1
  Logical Operator1/1 -> Logical Operator2/2
  Logical Operator5/1 -> Gain2/1
  Data Type Conversion1/1 -> Mux/2
  Fcn1/1 -> Relational Operator9/2, Relational Operator6/2
  Fcn3/1 -> Relational Operator12/2, Relational Operator7/2
  Logical Operator3/1 -> Logical Operator4/2
  Fcn4/1 -> Relational Operator8/2, Relational Operator4/2
  Fcn6/1 -> Relational Operator2/2
  Gain2/1 -> Data Type Conversion2/1
  Logical Operator2/1 -> Gain/1
  V12-07/1 -> Fcn1/1, Fcn4/1, Fcn6/1, Fcn5/1, Fcn3/1, Fcn2/1, Fcn/1
  Fcn2/1 -> Relational Operator11/2, Relational Operator10/2
  Fcn5/1 -> Relational Operator5/2, Relational Operator1/2
  Gain3/1 -> Data Type Conversion3/1
  Mux/1 -> Output/1
  Data Type Conversion2/1 -> Mux/3
  Relational Operator7/1 -> Logical Operator6/1
  Data Type Conversion/1 -> Mux/1
  Relational Operator6/1 -> Logical Operator7/2
  Relational Operator3/1 -> Logical Operator7/1
  Logical Operator7/1 -> Logical Operator4/1
  Relational Operator10/1 -> Logical Operator8/2
  Gain1/1 -> Data Type Conversion1/1
  Logical Operator9/1 -> Gain3/1
  Relational Operator/1 -> Logical Operator2/1
  Relational Operator1/1 -> Logical Operator1/1
  Relational Operator2/1 -> Logical Operator1/2
  Gain/1 -> Data Type Conversion/1
